simulink model "TEST_TCP"  (R2022b)
settings: Solver=FixedStepAuto  StartTime=0.0  StopTime=inf  FixedStep=1e-3  RelTol=1e-3  EnableMultiTasking=on
undefined symbols (not defined in the file or in its folder): angular, CIRCUIT, CLTF_DAMP, CLTF_FREQ, CLTF_GAIN, CONTROL, CONTROL_INI, DiscIntNeverNeededParam, INPUT, linear, MCP3201, MD25, MODEL, MODEL_INI, mpcstate, MPU60X0, MPU9250, MSG, NAV_MPC_CONTROL, OUTPUT, RCRX, SAMPLING_TIME, SYSID_INPUT, VL6180X
libraries: raspberrypiCommlib x156, simulink x86, dspsigattribs x14, raspberrypiNetworklib x13, embedlinuxBasiclib x9, ctrlSharedLib x2, ros2lib x2, mpclib x1, vrlib x1, sldrtlib x1
(part 3 of 17)

== system TEST_TCP/SIMULATION/READ IMU ==
  " LPF 3" : Subsystem
  " LPF 4" : Subsystem
  ACCEL_X : RandomNumber  Variance=MODEL_INI.PARAM.IMU_ACCEL_NOISE^2  Seed=500  SampleTime=MPU60X0.SAMPLING_TIME
  ACCEL_Y : RandomNumber  Variance=MODEL_INI.PARAM.IMU_ACCEL_NOISE^2  Seed=1000  SampleTime=MPU60X0.SAMPLING_TIME
  ACCEL_Z : RandomNumber  Variance=MODEL_INI.PARAM.IMU_ACCEL_NOISE^2  Seed=2000  SampleTime=MPU60X0.SAMPLING_TIME
  Bus Selector : BusSelector  OutputSignals=OUTPUT.matDCM_BE,OUTPUT.BODY_VEL_DER,OUTPUT.BODY_RATE_DER,OUTPUT.BODY_RATE
  Constant : Constant  Value=[0 0 -MODEL_INI.PARAM.GRAVITY]'  SampleTime=MPU60X0.SAMPLING_TIME
  Constant3 : Constant  Value=CONTROL_INI.PARAM.GRAVITY  SampleTime=MPU60X0.SAMPLING_TIME
  Constant5 : Constant  Value=MPU60X0.ACCEL_CALIB  SampleTime=MPU60X0.SAMPLING_TIME
  Constant6 : Constant  Value=MPU60X0.ALFA_CALIB  SampleTime=MPU60X0.SAMPLING_TIME
  Data Store Memory1 : DataStoreMemory  Priority=10  DataStoreName=MPU60X0_PITCH_OFFS  ReadBeforeWriteMsg=warning  WriteAfterWriteMsg=warning  WriteAfterReadMsg=warning  ShowAdditionalParam=off  OutDataTypeStr=double
  Data Store Memory3 : DataStoreMemory  Priority=10  DataStoreName=MPU60X0_ACCEL_OFFS  ReadBeforeWriteMsg=warning  WriteAfterWriteMsg=warning  WriteAfterReadMsg=warning  InitialValue=zeros(3,1)  ShowAdditionalParam=off  OutDataTypeStr=double
  Data Store Memory4 : DataStoreMemory  Priority=10  DataStoreName=MPU60X0_GYRO_OFFS  ReadBeforeWriteMsg=warning  WriteAfterWriteMsg=warning  WriteAfterReadMsg=warning  InitialValue=zeros(3,1)  ShowAdditionalParam=off  OutDataTypeStr=double
  Data Store Read : DataStoreRead  DataStoreName=CONTROL  DataStoreElements=CONTROL.STATE.VEHICLE_MODE  IndexOptions=Index vector (dialog)  Indices=1  OutputSizes=1
  Data Store Read1 : DataStoreRead  DataStoreName=MPU60X0_ACCEL_OFFS  SampleTime=MPU60X0.SAMPLING_TIME  IndexOptions=Index vector (dialog)  Indices=1  OutputSizes=1
  Data Store Read10 : DataStoreRead  DataStoreName=MODEL  SampleTime=MPU60X0.SAMPLING_TIME  IndexOptions=Index vector (dialog)  Indices=1  OutputSizes=1
  Data Store Read12 : DataStoreRead  DataStoreName=CONTROL  SampleTime=MPU60X0.SAMPLING_TIME  IndexOptions=Index vector (dialog)  Indices=1  OutputSizes=1
  Data Store Read2 : DataStoreRead  DataStoreName=MPU60X0_PITCH_OFFS  SampleTime=MPU60X0.SAMPLING_TIME  IndexOptions=Index vector (dialog)  Indices=1  OutputSizes=1
  Data Store Read4 : DataStoreRead  DataStoreName=MPU60X0_GYRO_OFFS  SampleTime=MPU60X0.SAMPLING_TIME  IndexOptions=Index vector (dialog)  Indices=1  OutputSizes=1
  Data Store Write : DataStoreWrite  DataStoreName=MPU60X0_ACCEL_OFFS  IndexOptions=Index vector (dialog)  Indices=1  OutputSizes=1
  Data Store Write1 : DataStoreWrite  DataStoreName=MPU60X0_GYRO_OFFS  IndexOptions=Index vector (dialog)  Indices=1  OutputSizes=1
  Data Store Write5 : DataStoreWrite  DataStoreName=CONTROL  IndexOptions=Index vector (dialog)  Indices=1  OutputSizes=1
  Divide : Product  Inputs=**  Multiplication=Matrix(*)
  FILTER POLE : Subsystem
  GRAVITY ROTATION : MATLAB Function  TreatAsAtomicUnit=on
  GYRO_X : RandomNumber  Variance=MODEL_INI.PARAM.IMU_GYRO_NOISE^2  Seed=3000  SampleTime=MPU60X0.SAMPLING_TIME
  GYRO_Y : RandomNumber  Variance=MODEL_INI.PARAM.IMU_GYRO_NOISE^2  Seed=4000  SampleTime=MPU60X0.SAMPLING_TIME
  GYRO_Z : RandomNumber  Variance=MODEL_INI.PARAM.IMU_GYRO_NOISE^2  Seed=5000  SampleTime=MPU60X0.SAMPLING_TIME
  Gain1 : Gain  Gain=MODEL_INI.PARAM.NOISE_FLAG
  Gain2 : Gain  Gain=MODEL_INI.PARAM.NOISE_FLAG
  IMU CALIBRATION : MATLAB Function  Priority=30  TreatAsAtomicUnit=on
  LPF 1 : Subsystem
  LPF 2 2 : Subsystem
  MEAN FILTER : DiscreteFilter  Numerator=1/floor(SAMPLING_TIME*1000)*ones(1,floor(SAMPLING_TIME*1000))  Denominator=[1 zeros(1,floor(SAMPLING_TIME*1000)-1)]
  "MEAN FILTER " : DiscreteFilter  Numerator=1/floor(SAMPLING_TIME*1000)*ones(1,floor(SAMPLING_TIME*1000))  Denominator=[1 zeros(1,floor(SAMPLING_TIME*1000)-1)]
  Math Function : Math  Operator=transpose  SignedPower=on
  Mux : Mux  Inputs=3
  Mux1 : Mux  Inputs=3
  Sum : Sum
  Sum1 : Sum  Inputs=++|
  Sum2 : Sum  Inputs=++|
  Terminator : Terminator
  wires:
  Sum1/1 -> IMU CALIBRATION/2(ACCEL), LPF 1/1(IN), MEAN FILTER/1
  MEAN FILTER/1 -> IMU CALIBRATION/4(ACCEL_MEAN), LPF 2 2/1(IN)
  IMU CALIBRATION/2(ACCEL_OFFS_OUT) -> Data Store Write/1
  Sum2/1 -> IMU CALIBRATION/6(GYRO), " LPF 3"/1(IN), "MEAN FILTER "/1
  IMU CALIBRATION/3(GYRO_OFFS_OUT) -> Data Store Write1/1
  Constant5/1 -> IMU CALIBRATION/10(ACCEL_CALIB)
  Constant6/1 -> IMU CALIBRATION/11(ALFA_CALIB)
  "MEAN FILTER "/1 -> IMU CALIBRATION/8(GYRO_MEAN), " LPF 4"/1(IN)
  " LPF 4"/1(OUT) -> IMU CALIBRATION/9(GYRO_MEAN_FILT)
  LPF 2 2/1(OUT) -> IMU CALIBRATION/5(ACCEL_MEAN_FILT)
  Data Store Read12/1 -> IMU CALIBRATION/1(CONTROL_IN)
  IMU CALIBRATION/1(CONTROL) -> Data Store Write5/1
  Mux/1 -> Gain2/1  "GYRO_NOISE"
  ACCEL_X/1 -> Mux1/1
  ACCEL_Y/1 -> Mux1/2
  Mux1/1 -> Gain1/1  "ACCEL_NOISE"
  GYRO_Z/1 -> Mux/3
  ACCEL_Z/1 -> Mux1/3
  GYRO_X/1 -> Mux/1
  GYRO_Y/1 -> Mux/2
  Data Store Read10/1 -> Bus Selector/1
  Bus Selector/1 -> Math Function/1  "<matDCM_BE>"
  Constant/1 -> Divide/2
  Divide/1 -> Sum/1
  Math Function/1 -> Divide/1
  Sum/1 -> Sum1/2
  Bus Selector/4 -> Sum2/1  "<BODY_RATE>"
  Data Store Read1/1 -> IMU CALIBRATION/12(ACCEL_OFFS_IN)
  Data Store Read4/1 -> IMU CALIBRATION/13(GYRO_OFFS_IN)
  Gain2/1 -> Sum2/2
  Bus Selector/2 -> Sum/2  "<BODY_VEL_DER>"
  Bus Selector/3 -> Terminator/1  "<BODY_RATE_DER>"
  FILTER POLE/1(ALFA) -> " LPF 4"/2(ALFA), " LPF 3"/2(ALFA), LPF 1/2(ALFA), LPF 2 2/2(ALFA)
  GRAVITY ROTATION/1(GRAVITY_VECTOR) -> IMU CALIBRATION/14(GRAVITY_VECTOR)
  LPF 1/1(OUT) -> IMU CALIBRATION/3(ACCEL_FILT)
  " LPF 3"/1(OUT) -> IMU CALIBRATION/7(GYRO_FILT)
  Constant3/1 -> GRAVITY ROTATION/2(GRAVITY)
  Data Store Read/1 -> GRAVITY ROTATION/3(VEHICLE_MODE)
  Data Store Read2/1 -> GRAVITY ROTATION/1(PITCH_OFFSET)
  Gain1/1 -> Sum1/1

== system TEST_TCP/CONTROL/LOCAL TARGETS/FORWARD VELOCITY TARGET ==
  Enable : EnablePort
  " PULSE GENERATION" : MATLAB Function  Priority=60  TreatAsAtomicUnit=on
  Bias : Bias  Bias=1  SaturateOnIntegerOverflow=off
  Cast1 : DataTypeConversion  OutDataTypeStr=double  SaturateOnIntegerOverflow=off  RndMeth=Floor
  Compare To Constant : simulink/Logic and Bit Operations/Compare To Constant  relop===  const=0  OutDataTypeStr=boolean
  Compare To Constant1 : simulink/Logic and Bit Operations/Compare To Constant  relop=>=  const=5  OutDataTypeStr=boolean
  Constant : Constant  Value=SYSID_INPUT(:,1)  SampleTime=SAMPLING_TIME
  Constant1 : Constant  Value=0  OutDataTypeStr=double  SampleTime=SAMPLING_TIME
  Constant2 : Constant  Value=0.15  OutDataTypeStr=double  SampleTime=SAMPLING_TIME
  Constant3 : Constant  Value=SAMPLING_TIME  OutDataTypeStr=double  SampleTime=SAMPLING_TIME
  Constant5 : Constant  Value=0.25  OutDataTypeStr=double  SampleTime=SAMPLING_TIME
  Counter Free-Running : simulink/Sources/Counter Free-Running  NumBits=9  tsamp=SAMPLING_TIME
  Data Store Read : DataStoreRead  DataStoreName=CONTROL  SampleTime=SAMPLING_TIME  DataStoreElements=CONTROL.STATE.FV_TARGET_TYPE  IndexOptions=Index vector (dialog)  Indices=1  OutputSizes=1
  Data Store Read1 : DataStoreRead  DataStoreName=CONTROL  SampleTime=SAMPLING_TIME  DataStoreElements=CONTROL.PARAM.OP_OUTPUT(1,:)#CONTROL.PARAM.FV_TARGET_VALUE  IndexOptions=Index vector (dialog)  Indices=1  OutputSizes=1
  Data Store Read2 : DataStoreRead  DataStoreName=CONTROL  SampleTime=SAMPLING_TIME  DataStoreElements=CONTROL.PARAM.OP_OUTPUT(1,:)  IndexOptions=Index vector (dialog)  Indices=1  OutputSizes=1
  Data Store Read3 : DataStoreRead  DataStoreName=CONTROL  SampleTime=SAMPLING_TIME  IndexOptions=Index vector (dialog)  Indices=1  OutputSizes=1
  Data Store Read4 : DataStoreRead  DataStoreName=CONTROL  SampleTime=SAMPLING_TIME  DataStoreElements=CONTROL.STATE.FV_TARGET_TYPE  IndexOptions=Index vector (dialog)  Indices=1  OutputSizes=1
  Data Store Read5 : DataStoreRead  DataStoreName=CONTROL  SampleTime=SAMPLING_TIME  DataStoreElements=CONTROL.PARAM.SAMPLING_TIME  IndexOptions=Index vector (dialog)  Indices=1  OutputSizes=1
  Data Store Read6 : DataStoreRead  DataStoreName=CONTROL  SampleTime=SAMPLING_TIME  DataStoreElements=CONTROL.STATE.VEHICLE_MODE  IndexOptions=Index vector (dialog)  Indices=1  OutputSizes=1
  Data Store Read7 : DataStoreRead  DataStoreName=CONTROL  SampleTime=SAMPLING_TIME  DataStoreElements=CONTROL.STATE.VEHICLE_MODE  IndexOptions=Index vector (dialog)  Indices=1  OutputSizes=1
  Data Store Write1 : DataStoreWrite  DataStoreName=CONTROL  SampleTime=SAMPLING_TIME  DataStoreElements=CONTROL.TARGET.FORWARD_VEL_REF_LC  IndexOptions=Index vector (dialog)  Indices=1  OutputSizes=1
  Data Type Conversion : DataTypeConversion  OutDataTypeStr=double  SaturateOnIntegerOverflow=off  RndMeth=Floor
  Gain2 : Gain  Gain=0.15/2
  Logical Operator : Logic  Operator=OR  AllPortsSameDT=off  OutDataTypeStr=boolean
  Multiport Switch : MultiPortSwitch  DataPortOrder=Zero-based contiguous  Inputs=6  zeroidx=on  SaturateOnIntegerOverflow=off  InputSameDT=off
  Mux : Mux  Inputs=2
  Product : Product
  Pulse Generator1 : DiscretePulseGenerator  Amplitude=0.15  Period=round(10/SAMPLING_TIME)  PulseWidth=round(5/SAMPLING_TIME)  SampleTime=SAMPLING_TIME
  Pulse Generator2 : DiscretePulseGenerator  Amplitude=0.15  Period=round(3/SAMPLING_TIME)  PulseWidth=round(1.5/SAMPLING_TIME)  PhaseDelay=round(0/SAMPLING_TIME)  SampleTime=SAMPLING_TIME
  RAMP : MATLAB Function  TreatAsAtomicUnit=on
  Selector : Selector  IndexMode=Zero-based  InputPortWidth=512  IndexOptions=Index vector (port)  Indices=[1 3]  OutputSizes=1
  Selector1 : Selector  IndexMode=Zero-based  InputPortWidth=5  IndexOptions=Index vector (port)  Indices=[1 3]  OutputSizes=1
  Selector2 : Selector  InputPortWidth=4  IndexOptions=Index vector (port)  Indices=[1 3]  OutputSizes=1
  Sum1 : Sum  Inputs=|++
  Sum3 : Sum  Inputs=|++
  Sum6 : Sum  Inputs=|++
  Switch : Switch  Criteria=u2 > Threshold  Threshold=0.5  SaturateOnIntegerOverflow=off  InputSameDT=off
  Unit Delay : UnitDelay  SampleTime=SAMPLING_TIME  HasFrameUpgradeWarning=on
  wires:
  Constant5/1 -> Sum3/2
  Counter Free-Running/1 -> Cast1/1
  Sum6/1 -> Multiport Switch/5
  Gain2/1 -> Sum6/1
  Selector1/1 -> Multiport Switch/2
  Constant/1 -> Selector/1
  Data Store Read/1 -> Multiport Switch/1
  Cast1/1 -> Selector/2
  Constant2/1 -> Sum6/2
  Multiport Switch/1 -> Data Store Write1/1
  Data Store Read3/1 -> " PULSE GENERATION"/1(CONTROL)
  " PULSE GENERATION"/1(FORWARD_VEL_REF) -> Multiport Switch/3
  Data Store Read1/2 -> Selector1/2
  Selector2/1 -> Multiport Switch/6
  Data Store Read2/1 -> Selector2/1
  Data Store Read4/1 -> Multiport Switch/7
  RAMP/1(ramp_out) -> Selector2/2
  Data Store Read5/1 -> RAMP/1(SAMPLING_TIME)
  Selector/1 -> Bias/1
  Bias/1 -> Gain2/1
  Mux/1 -> Selector1/1
  Data Store Read1/1 -> Mux/2
  Constant1/1 -> Mux/1
  Sum3/1 -> Product/2
  Product/1 -> Multiport Switch/4
  Compare To Constant/1 -> Logical Operator/1
  Data Store Read6/1 -> Compare To Constant/1
  Logical Operator/1 -> Product/1
  Unit Delay/1 -> Sum1/2
  Constant3/1 -> Sum1/1
  Compare To Constant1/1 -> Logical Operator/2
  Sum1/1 -> Compare To Constant1/1, Unit Delay/1
  Data Store Read7/1 -> Data Type Conversion/1
  Switch/1 -> Sum3/1
  Pulse Generator2/1 -> Switch/3
  Pulse Generator1/1 -> Switch/1
  Data Type Conversion/1 -> Switch/2

== system TEST_TCP/CONTROL/LOCAL TARGETS/NAVIGATION TARGETS ==
  Enable : EnablePort
  Constant : Constant  SampleTime=SAMPLING_TIME
  Constant1 : Constant  SampleTime=SAMPLING_TIME
  Data Store Read : DataStoreRead  DataStoreName=CONTROL  SampleTime=SAMPLING_TIME  DataStoreElements=CONTROL.STATE.NAV_TARGET_TYPE(1,1)  IndexOptions=Index vector (dialog)  Indices=1  OutputSizes=1
  Data Store Read2 : DataStoreRead  DataStoreName=CONTROL  SampleTime=SAMPLING_TIME  DataStoreElements=CONTROL.STATE.NAV_TARGET_TYPE(1,2)  IndexOptions=Index vector (dialog)  Indices=1  OutputSizes=1
  Data Store Read4 : DataStoreRead  DataStoreName=CONTROL  SampleTime=SAMPLING_TIME  DataStoreElements=CONTROL.PARAM.NAV_TARGET_VALUE(1,2)  IndexOptions=Index vector (dialog)  Indices=1  OutputSizes=1
  Data Store Read7 : DataStoreRead  Commented=on  DataStoreName=CONTROL  SampleTime=SAMPLING_TIME  IndexOptions=Index vector (dialog)  Indices=1  OutputSizes=1
  Data Store Read9 : DataStoreRead  DataStoreName=CONTROL  SampleTime=SAMPLING_TIME  DataStoreElements=CONTROL.PARAM.NAV_TARGET_VALUE(1,1)  IndexOptions=Index vector (dialog)  Indices=1  OutputSizes=1
  Data Store Write : DataStoreWrite  Commented=on  DataStoreName=CONTROL  SampleTime=SAMPLING_TIME  IndexOptions=Index vector (dialog)  Indices=1  OutputSizes=1
  Data Store Write1 : DataStoreWrite  DataStoreName=CONTROL  SampleTime=SAMPLING_TIME  DataStoreElements=CONTROL.TARGET.NAV_REF_LC(1,1)  IndexOptions=Index vector (dialog)  Indices=1  OutputSizes=1
  Data Store Write2 : DataStoreWrite  DataStoreName=CONTROL  SampleTime=SAMPLING_TIME  DataStoreElements=CONTROL.TARGET.NAV_REF_LC(2,1)  IndexOptions=Index vector (dialog)  Indices=1  OutputSizes=1
  Multiport Switch : MultiPortSwitch  DataPortOrder=Zero-based contiguous  Inputs=4  zeroidx=on  SaturateOnIntegerOverflow=off  InputSameDT=off
  Multiport Switch1 : MultiPortSwitch  DataPortOrder=Zero-based contiguous  Inputs=4  zeroidx=on  SaturateOnIntegerOverflow=off  InputSameDT=off
  PATH PLANNER : MATLAB Function  Priority=10  Commented=on  TreatAsAtomicUnit=on
  Pulse Generator1 : DiscretePulseGenerator  Amplitude=2  Period=round(50/SAMPLING_TIME)  PulseWidth=round(25/SAMPLING_TIME)  PhaseDelay=round(12.5/SAMPLING_TIME)  SampleTime=SAMPLING_TIME
  Pulse Generator2 : DiscretePulseGenerator  Amplitude=2  Period=round(50/SAMPLING_TIME)  PulseWidth=round(25/SAMPLING_TIME)  SampleTime=SAMPLING_TIME
  Sine Wave : Sin  SineType=Sample based  Samples=round(40/SAMPLING_TIME)  SampleTime=SAMPLING_TIME
  Sine Wave1 : Sin  SineType=Sample based  Samples=round(40/SAMPLING_TIME)  SampleTime=SAMPLING_TIME  Offset=round(30/SAMPLING_TIME)
  Sum1 : Sum  Inputs=|+-
  Sum3 : Sum  Inputs=|+-
  TRAJECTORY PLANNER (POLYNOMIAL IN Vx & Vy) : MATLAB Function  Priority=10  Commented=on  TreatAsAtomicUnit=on
  wires:
  Data Store Read7/1 -> TRAJECTORY PLANNER (POLYNOMIAL IN Vx & Vy)/1(CONTROL_IN)
  TRAJECTORY PLANNER (POLYNOMIAL IN Vx & Vy)/1(CONTROL) -> Data Store Write/1
  Data Store Read/1 -> Multiport Switch/1
  Multiport Switch/1 -> Data Store Write1/1
  Sum3/1 -> Multiport Switch/5, Multiport Switch/3
  Data Store Read9/1 -> Multiport Switch/2
  Sine Wave/1 -> Multiport Switch/4
  Data Store Read4/1 -> Multiport Switch1/2
  Data Store Read2/1 -> Multiport Switch1/1
  Sine Wave1/1 -> Multiport Switch1/4
  Multiport Switch1/1 -> Data Store Write2/1
  Sum1/1 -> Multiport Switch1/5, Multiport Switch1/3
  Pulse Generator2/1 -> Sum3/1
  Constant/1 -> Sum3/2
  Pulse Generator1/1 -> Sum1/1
  Constant1/1 -> Sum1/2

== system TEST_TCP/CONTROL/LOCAL TARGETS/OPL TARGETS ==
  Enable : EnablePort
  Cast : DataTypeConversion  OutDataTypeStr=uint8  SaturateOnIntegerOverflow=off  RndMeth=Floor
  Cast1 : DataTypeConversion  OutDataTypeStr=double  SaturateOnIntegerOverflow=off  RndMeth=Floor
  Constant : Constant  Value=SYSID_INPUT(:,1)  SampleTime=SAMPLING_TIME
  Constant1 : Constant  Value=SYSID_INPUT(:,2)  SampleTime=SAMPLING_TIME
  Constant2 : Constant  Value=2  OutDataTypeStr=single  SampleTime=SAMPLING_TIME
  Constant3 : Constant  Value=2  OutDataTypeStr=double  SampleTime=SAMPLING_TIME
  Constant5 : Constant  Value=4  OutDataTypeStr=double  SampleTime=SAMPLING_TIME
  Constant6 : Constant  Value=0  OutDataTypeStr=double  SampleTime=SAMPLING_TIME
  Constant7 : Constant  Value=-0.25  OutDataTypeStr=single  SampleTime=SAMPLING_TIME
  Constant8 : Constant  Value=2  OutDataTypeStr=double  SampleTime=SAMPLING_TIME
  Counter Free-Running : simulink/Sources/Counter Free-Running  NumBits=9  tsamp=SAMPLING_TIME
  Counter Free-Running1 : simulink/Sources/Counter Free-Running  NumBits=9  tsamp=SAMPLING_TIME
  Data Store Read : DataStoreRead  DataStoreName=CONTROL  SampleTime=SAMPLING_TIME  DataStoreElements=CONTROL.STATE.MV_TARGET_TYPE(1,1)  IndexOptions=Index vector (dialog)  Indices=1  OutputSizes=1
  Data Store Read1 : DataStoreRead  DataStoreName=CONTROL  SampleTime=SAMPLING_TIME  IndexOptions=Index vector (dialog)  Indices=1  OutputSizes=1
  Data Store Read2 : DataStoreRead  DataStoreName=CONTROL  SampleTime=SAMPLING_TIME  DataStoreElements=CONTROL.STATE.MV_TARGET_TYPE(2,1)  IndexOptions=Index vector (dialog)  Indices=1  OutputSizes=1
  Data Store Write1 : DataStoreWrite  DataStoreName=CONTROL  SampleTime=SAMPLING_TIME  DataStoreElements=CONTROL.TARGET.MOTOR_VOLT_CD_REF_LC(:,:)  IndexOptions=Index vector (dialog)  Indices=1  OutputSizes=1
  Gain2 : Gain
  Gain3 : Gain
  Multiport Switch : MultiPortSwitch  DataPortOrder=Zero-based contiguous  Inputs=4  zeroidx=on  SaturateOnIntegerOverflow=off  InputSameDT=off
  Multiport Switch1 : MultiPortSwitch  DataPortOrder=Zero-based contiguous  Inputs=4  zeroidx=on  SaturateOnIntegerOverflow=off  InputSameDT=off
  Mux : Mux  Inputs=2
  Pulse Generator1 : DiscretePulseGenerator  Amplitude=2  Period=200  PulseWidth=100  SampleTime=SAMPLING_TIME
  Pulse Generator3 : DiscretePulseGenerator  Amplitude=2  Period=200  PulseWidth=100  SampleTime=SAMPLING_TIME
  Selector : Selector  IndexMode=Zero-based  InputPortWidth=512  IndexOptions=Index vector (port)  Indices=[1 3]  OutputSizes=1
  Selector1 : Selector  IndexMode=Zero-based  InputPortWidth=512  IndexOptions=Index vector (port)  Indices=[1 3]  OutputSizes=1
  Sum{1,3,6,8} (4 alike) : Sum  Inputs=|++
  VOLTAGE PULSE GENERATION : MATLAB Function  Priority=60  TreatAsAtomicUnit=on
  wires:
  VOLTAGE PULSE GENERATION/1(MOTOR_VOLT_TARGET) -> Multiport Switch/3, Multiport Switch1/3
  Constant6/1 -> Multiport Switch1/2
  Constant7/1 -> Sum8/2
  Sum6/1 -> Multiport Switch/5
  Mux/1 -> Data Store Write1/1
  Sum3/1 -> Multiport Switch/4
  Gain2/1 -> Sum6/1
  Counter Free-Running/1 -> Cast1/1
  Cast1/1 -> Selector/2
  Sum8/1 -> Multiport Switch1/5
  Sum1/1 -> Multiport Switch1/4
  Selector1/1 -> Gain3/1
  Multiport Switch1/1 -> Mux/2
  Constant1/1 -> Selector1/1
  Constant/1 -> Selector/1
  Gain3/1 -> Sum8/1
  Multiport Switch/1 -> Mux/1
  Data Store Read2/1 -> Multiport Switch1/1
  Cast/1 -> Selector1/2
  Constant2/1 -> Sum6/2
  Selector/1 -> Gain2/1
  Counter Free-Running1/1 -> Cast/1
  Data Store Read/1 -> Multiport Switch/1
  Data Store Read1/1 -> VOLTAGE PULSE GENERATION/1(CONTROL)
  Constant5/1 -> Multiport Switch/2
  Pulse Generator1/1 -> Sum3/1
  Constant3/1 -> Sum3/2
  Pulse Generator3/1 -> Sum1/1
  Constant8/1 -> Sum1/2

== system TEST_TCP/CONTROL/LOCAL TARGETS/WFL TARGETS ==
  Enable : EnablePort
  " PULSE GENERATION" : MATLAB Function  Priority=60  TreatAsAtomicUnit=on
  Cast1 : DataTypeConversion  OutDataTypeStr=double  SaturateOnIntegerOverflow=off  RndMeth=Floor
  Compare To Constant : simulink/Logic and Bit Operations/Compare To Constant  relop=<=  const=3.0  OutDataTypeStr=uint8
  Constant : Constant  Value=SYSID_INPUT(:,1)  SampleTime=SAMPLING_TIME
  Constant1 : Constant  Value=0.1  OutDataTypeStr=double  SampleTime=SAMPLING_TIME
  Constant3 : Constant  Value=0.25  OutDataTypeStr=double  SampleTime=SAMPLING_TIME
  Constant5 : Constant  Value=0.025  OutDataTypeStr=single  SampleTime=SAMPLING_TIME
  Counter Free-Running : simulink/Sources/Counter Free-Running  NumBits=9  tsamp=SAMPLING_TIME
  Data Store Read : DataStoreRead  DataStoreName=CONTROL  SampleTime=SAMPLING_TIME  DataStoreElements=CONTROL.STATE.WD_TARGET_TYPE  IndexOptions=Index vector (dialog)  Indices=1  OutputSizes=1
  Data Store Read1 : DataStoreRead  DataStoreName=CONTROL  SampleTime=SAMPLING_TIME  DataStoreElements=CONTROL.STATE.WALL_FOLLOWER_MODE  IndexOptions=Index vector (dialog)  Indices=1  OutputSizes=1
  Data Store Read3 : DataStoreRead  DataStoreName=CONTROL  SampleTime=SAMPLING_TIME  IndexOptions=Index vector (dialog)  Indices=1  OutputSizes=1
  Data Store Write1 : DataStoreWrite  DataStoreName=CONTROL  SampleTime=SAMPLING_TIME  DataStoreElements=CONTROL.TARGET.WALL_DIST_REF_LC  IndexOptions=Index vector (dialog)  Indices=1  OutputSizes=1
  Data Type Conversion : DataTypeConversion  OutDataTypeStr=double  SaturateOnIntegerOverflow=off  RndMeth=Floor
  Gain2 : Gain  Gain=0.025
  Multiport Switch : MultiPortSwitch  DataPortOrder=Zero-based contiguous  Inputs=4  zeroidx=on  SaturateOnIntegerOverflow=off  InputSameDT=off
  Product : Product
  Pulse Generator1 : DiscretePulseGenerator  Amplitude=0.025  Period=1000  PulseWidth=500  SampleTime=SAMPLING_TIME
  Selector : Selector  IndexMode=Zero-based  InputPortWidth=512  IndexOptions=Index vector (port)  Indices=[1 3]  OutputSizes=1
  Sum3 : Sum  Inputs=+|+|-
  Sum6 : Sum  Inputs=|++
  Switch : Switch  Criteria=u2 > Threshold  Threshold=0.5  SaturateOnIntegerOverflow=off  InputSameDT=off
  wires:
  Data Store Read3/1 -> " PULSE GENERATION"/1(CONTROL)
  Sum6/1 -> Multiport Switch/5
  Sum3/1 -> Multiport Switch/4
  Constant/1 -> Selector/1
  " PULSE GENERATION"/1(WALL_DIST_REF) -> Multiport Switch/3
  Switch/1 -> Sum6/2, Sum3/1, Multiport Switch/2
  Gain2/1 -> Sum6/1
  Multiport Switch/1 -> Data Store Write1/1
  Cast1/1 -> Selector/2
  Selector/1 -> Gain2/1
  Counter Free-Running/1 -> Cast1/1
  Product/1 -> Multiport Switch/1
  Data Store Read/1 -> Compare To Constant/1, Product/1
  Compare To Constant/1 -> Product/2
  Constant3/1 -> Switch/1
  Constant1/1 -> Switch/3
  Pulse Generator1/1 -> Sum3/2
  Constant5/1 -> Sum3/3
  Data Store Read1/1 -> Data Type Conversion/1
  Data Type Conversion/1 -> Switch/2

== system TEST_TCP/CONTROL/LOCAL TARGETS/YAW ANGLE TARGET ==
  Enable : EnablePort
  " PULSE GENERATION" : MATLAB Function  Priority=60  TreatAsAtomicUnit=on
  Cast1 : DataTypeConversion  OutDataTypeStr=double  SaturateOnIntegerOverflow=off  RndMeth=Floor
  Constant : Constant  Value=SYSID_INPUT(:,1)  SampleTime=SAMPLING_TIME
  Constant3 : Constant  Value=0  OutDataTypeStr=double  SampleTime=SAMPLING_TIME
  Constant5 : Constant  Value=-60*pi/180  OutDataTypeStr=single  SampleTime=SAMPLING_TIME
  Constant8 : Constant  Value=-60*pi/180  OutDataTypeStr=single  SampleTime=SAMPLING_TIME
  Counter Free-Running : simulink/Sources/Counter Free-Running  NumBits=9  tsamp=SAMPLING_TIME
  Data Store Read : DataStoreRead  DataStoreName=CONTROL  SampleTime=SAMPLING_TIME  DataStoreElements=CONTROL.STATE.YA_TARGET_TYPE  IndexOptions=Index vector (dialog)  Indices=1  OutputSizes=1
  Data Store Read1 : DataStoreRead  DataStoreName=CONTROL  SampleTime=SAMPLING_TIME  IndexOptions=Index vector (dialog)  Indices=1  OutputSizes=1
  Data Store Write1 : DataStoreWrite  DataStoreName=CONTROL  SampleTime=SAMPLING_TIME  DataStoreElements=CONTROL.TARGET.YAW_ANG_REF_LC  IndexOptions=Index vector (dialog)  Indices=1  OutputSizes=1
  Gain2 : Gain  Gain=120*pi/180
  Multiport Switch : MultiPortSwitch  DataPortOrder=Zero-based contiguous  Inputs=4  zeroidx=on  SaturateOnIntegerOverflow=off  InputSameDT=off
  Pulse Generator1 : DiscretePulseGenerator  Amplitude=120*pi/180  Period=500  PulseWidth=250  PhaseDelay=125  SampleTime=SAMPLING_TIME
  Selector : Selector  IndexMode=Zero-based  InputPortWidth=512  IndexOptions=Index vector (port)  Indices=[1 3]  OutputSizes=1
  Sum3 : Sum  Inputs=|++
  Sum6 : Sum  Inputs=|++
  wires:
  Constant5/1 -> Sum3/2
  Selector/1 -> Gain2/1
  Pulse Generator1/1 -> Sum3/1
  Counter Free-Running/1 -> Cast1/1
  Sum6/1 -> Multiport Switch/5
  " PULSE GENERATION"/1(YAW_ANG_REF) -> Multiport Switch/3
  Sum3/1 -> Multiport Switch/4
  Gain2/1 -> Sum6/1
  Constant3/1 -> Multiport Switch/2
  Constant/1 -> Selector/1
  Data Store Read/1 -> Multiport Switch/1
  Data Store Read1/1 -> " PULSE GENERATION"/1(CONTROL)
  Cast1/1 -> Selector/2
  Constant8/1 -> Sum6/2
  Multiport Switch/1 -> Data Store Write1/1

== system TEST_TCP/CONTROL/LOCAL TARGETS/YAW RATE TARGET ==
  Enable : EnablePort
  " PULSE GENERATION " : MATLAB Function  Priority=60  TreatAsAtomicUnit=on
  Bias : Bias  Bias=1  SaturateOnIntegerOverflow=off
  Cast : DataTypeConversion  OutDataTypeStr=uint8  SaturateOnIntegerOverflow=off  RndMeth=Floor
  Constant1 : Constant  Value=SYSID_INPUT(:,2)  SampleTime=SAMPLING_TIME
  Constant6 : Constant  Value=0  OutDataTypeStr=double  SampleTime=SAMPLING_TIME
  Constant8 : Constant  Value=-60*pi/180  OutDataTypeStr=single  SampleTime=SAMPLING_TIME
  Constant9 : Constant  Value=-60*pi/180  OutDataTypeStr=single  SampleTime=SAMPLING_TIME
  Counter Free-Running1 : simulink/Sources/Counter Free-Running  NumBits=9  tsamp=SAMPLING_TIME
  Data Store Read1 : DataStoreRead  DataStoreName=CONTROL  SampleTime=SAMPLING_TIME  IndexOptions=Index vector (dialog)  Indices=1  OutputSizes=1
  Data Store Read2 : DataStoreRead  DataStoreName=CONTROL  SampleTime=SAMPLING_TIME  DataStoreElements=CONTROL.STATE.YR_TARGET_TYPE  IndexOptions=Index vector (dialog)  Indices=1  OutputSizes=1
  Data Store Write2 : DataStoreWrite  DataStoreName=CONTROL  SampleTime=SAMPLING_TIME  DataStoreElements=CONTROL.TARGET.YAW_RATE_REF_LC  IndexOptions=Index vector (dialog)  Indices=1  OutputSizes=1
  Gain1 : Gain  Gain=60*pi/180
  Multiport Switch1 : MultiPortSwitch  DataPortOrder=Zero-based contiguous  Inputs=4  zeroidx=on  SaturateOnIntegerOverflow=off  InputSameDT=off
  Pulse Generator2 : DiscretePulseGenerator  Amplitude=120*pi/180  Period=round(3/SAMPLING_TIME)  PulseWidth=round(1.5/SAMPLING_TIME)  PhaseDelay=round(0.75/SAMPLING_TIME)  SampleTime=SAMPLING_TIME
  Selector1 : Selector  IndexMode=Zero-based  InputPortWidth=512  IndexOptions=Index vector (port)  Indices=[1 3]  OutputSizes=1
  Sum1 : Sum  Inputs=|++
  Sum2 : Sum  Inputs=|++
  wires:
  Sum2/1 -> Multiport Switch1/5
  Data Store Read2/1 -> Multiport Switch1/1
  Constant1/1 -> Selector1/1
  Multiport Switch1/1 -> Data Store Write2/1
  Constant6/1 -> Multiport Switch1/2
  Counter Free-Running1/1 -> Cast/1
  Cast/1 -> Selector1/2
  Data Store Read1/1 -> " PULSE GENERATION "/1(CONTROL)
  " PULSE GENERATION "/1(YAW_RATE_REF) -> Multiport Switch1/3
  Constant8/1 -> Sum1/2
  Constant9/1 -> Sum2/2
  Pulse Generator2/1 -> Sum1/1
  Selector1/1 -> Bias/1
  Sum1/1 -> Multiport Switch1/4
  Gain1/1 -> Sum2/1
  Bias/1 -> Gain1/1

== system TEST_TCP/CONTROL/SYSTEM IDENTIFICATION/FILTER TIME CONSTANT ==
  Enable : EnablePort
  Constant5 : Constant  Value=0.05  OutDataTypeStr=single  SampleTime=SAMPLING_TIME
  Data Store Write1 : DataStoreWrite  DataStoreName=CONTROL  SampleTime=SAMPLING_TIME  DataStoreElements=CONTROL.PARAM.ENC_FILT_FREQ  IndexOptions=Index vector (dialog)  Indices=1  OutputSizes=1
  Data Store Write2 : DataStoreWrite  DataStoreName=CONTROL  SampleTime=SAMPLING_TIME  DataStoreElements=CONTROL.PARAM.FILT_TIME_CONSTANT_ACT  IndexOptions=Index vector (dialog)  Indices=1  OutputSizes=1
  Gain : Gain  Gain=1/2/pi
  Math Function : Math  Operator=reciprocal
  Pulse Generator1 : DiscretePulseGenerator  Amplitude=0.05  Period=16000  PulseWidth=8000  PhaseDelay=8000  SampleTime=SAMPLING_TIME
  Sum3 : Sum  Inputs=|++
  wires:
  Pulse Generator1/1 -> Sum3/1
  Constant5/1 -> Sum3/2
  Sum3/1 -> Data Store Write2/1, Math Function/1
  Math Function/1 -> Gain/1
  Gain/1 -> Data Store Write1/1

== system TEST_TCP/CONTROL/SYSTEM IDENTIFICATION/STATE VARIABLE FILTER 1 ==
  IN : Inport
  Add : Sum  Inputs=3
  Constant : Constant  Value=SVF_B1d  SampleTime=SAMPLING_TIME
  Constant1 : Constant  Value=SVF_B2d  SampleTime=SAMPLING_TIME
  Constant2 : Constant  Value=SVF_Ad  SampleTime=SAMPLING_TIME
  Divide : Product  Multiplication=Matrix(*)
  Divide1 : Product  Multiplication=Matrix(*)
  Divide2 : Product  Multiplication=Matrix(*)
  Unit Delay : UnitDelay  InitialCondition=zeros(4,1)  SampleTime=-1  HasFrameUpgradeWarning=on
  Unit Delay1 : UnitDelay  SampleTime=-1  HasFrameUpgradeWarning=on
  STATE : Outport  VectorParamsAs1DForOutWhenUnconnected=off
  wires:
  Constant/1 -> Divide1/1
  Unit Delay1/1 -> Divide1/2
  Divide1/1 -> Add/1
  Add/1 -> STATE/1, Unit Delay/1
  Divide/1 -> Add/2
  Constant1/1 -> Divide/1
  Divide2/1 -> Add/3
  Constant2/1 -> Divide2/1
  Unit Delay/1 -> Divide2/2
  IN/1 -> Divide/2, Unit Delay1/1

== system TEST_TCP/CONTROL/SYSTEM IDENTIFICATION/STATE VARIABLE FILTER 2 ==
  IN : Inport
  Add : Sum  Inputs=3
  Constant : Constant  Value=SVF_B1d  SampleTime=SAMPLING_TIME
  Constant1 : Constant  Value=SVF_B2d  SampleTime=SAMPLING_TIME
  Constant2 : Constant  Value=SVF_Ad  SampleTime=SAMPLING_TIME
  Divide : Product  Multiplication=Matrix(*)
  Divide1 : Product  Multiplication=Matrix(*)
  Divide2 : Product  Multiplication=Matrix(*)
  Unit Delay : UnitDelay  InitialCondition=zeros(4,1)  SampleTime=-1  HasFrameUpgradeWarning=on
  Unit Delay1 : UnitDelay  SampleTime=-1  HasFrameUpgradeWarning=on
  STATE : Outport  VectorParamsAs1DForOutWhenUnconnected=off
  wires:
  IN/1 -> Unit Delay1/1, Divide/2
  Unit Delay/1 -> Divide2/2
  Constant2/1 -> Divide2/1
  Divide2/1 -> Add/3
  Constant1/1 -> Divide/1
  Divide/1 -> Add/2
  Add/1 -> Unit Delay/1, STATE/1
  Divide1/1 -> Add/1
  Unit Delay1/1 -> Divide1/2
  Constant/1 -> Divide1/1

== system TEST_TCP/CONTROL/SYSTEM IDENTIFICATION/STATE VARIABLE FILTER 3 ==
  IN : Inport
  Add : Sum  Inputs=3
  Constant : Constant  Value=SVF_B1d  SampleTime=SAMPLING_TIME
  Constant1 : Constant  Value=SVF_B2d  SampleTime=SAMPLING_TIME
  Constant2 : Constant  Value=SVF_Ad  SampleTime=SAMPLING_TIME
  Divide : Product  Multiplication=Matrix(*)
  Divide1 : Product  Multiplication=Matrix(*)
  Divide2 : Product  Multiplication=Matrix(*)
  Unit Delay : UnitDelay  InitialCondition=zeros(4,1)  SampleTime=-1  HasFrameUpgradeWarning=on
  Unit Delay1 : UnitDelay  SampleTime=-1  HasFrameUpgradeWarning=on
  STATE : Outport  VectorParamsAs1DForOutWhenUnconnected=off
  wires:
  Constant/1 -> Divide1/1
  Unit Delay1/1 -> Divide1/2
  Divide1/1 -> Add/1
  Add/1 -> STATE/1, Unit Delay/1
  Divide/1 -> Add/2
  Constant1/1 -> Divide/1
  Divide2/1 -> Add/3
  Constant2/1 -> Divide2/1
  Unit Delay/1 -> Divide2/2
  IN/1 -> Divide/2, Unit Delay1/1

== system TEST_TCP/CONTROL/SYSTEM IDENTIFICATION/STATE VARIABLE FILTER 4 ==
  IN : Inport
  Add : Sum  Inputs=3
  Constant : Constant  Value=SVF_B1d  SampleTime=SAMPLING_TIME
  Constant1 : Constant  Value=SVF_B2d  SampleTime=SAMPLING_TIME
  Constant2 : Constant  Value=SVF_Ad  SampleTime=SAMPLING_TIME
  Divide : Product  Multiplication=Matrix(*)
  Divide1 : Product  Multiplication=Matrix(*)
  Divide2 : Product  Multiplication=Matrix(*)
  Unit Delay : UnitDelay  InitialCondition=zeros(4,1)  SampleTime=-1  HasFrameUpgradeWarning=on
  Unit Delay1 : UnitDelay  SampleTime=-1  HasFrameUpgradeWarning=on
  STATE : Outport  VectorParamsAs1DForOutWhenUnconnected=off
  wires:
  IN/1 -> Unit Delay1/1, Divide/2
  Unit Delay/1 -> Divide2/2
  Constant2/1 -> Divide2/1
  Divide2/1 -> Add/3
  Constant1/1 -> Divide/1
  Divide/1 -> Add/2
  Add/1 -> Unit Delay/1, STATE/1
  Divide1/1 -> Add/1
  Unit Delay1/1 -> Divide1/2
  Constant/1 -> Divide1/1

== system TEST_TCP/HARDWARE/ACTUATORS/MD25_I2C ==
  Cast : DataTypeConversion  OutDataTypeStr=uint8  SaturateOnIntegerOverflow=off  RndMeth=Floor
  Compare To Constant : simulink/Logic and Bit Operations/Compare To Constant  relop===  const=0  OutDataTypeStr=uint8
  Data Store Memory : DataStoreMemory  Priority=10  DataStoreName=MD25_INIT  ReadBeforeWriteMsg=warning  WriteAfterWriteMsg=warning  WriteAfterReadMsg=warning  ShowAdditionalParam=off  OutDataTypeStr=boolean
  Data Store Read : DataStoreRead  DataStoreName=MD25_INIT  SampleTime=SAMPLING_TIME  IndexOptions=Index vector (dialog)  Indices=1  OutputSizes=1
  Data Store Read1 : DataStoreRead  DataStoreName=MD25_INIT  IndexOptions=Index vector (dialog)  Indices=1  OutputSizes=1
  Data Store Read2 : DataStoreRead  DataStoreName=CONTROL  SampleTime=SAMPLING_TIME  DataStoreElements=CONTROL.STATE.CURRENT_STATUS_SYS  IndexOptions=Index vector (dialog)  Indices=1  OutputSizes=1
  Data Store Write : DataStoreWrite  DataStoreName=CONTROL  DataStoreElements=CONTROL.STATE.MD25_INIT  IndexOptions=Index vector (dialog)  Indices=1  OutputSizes=1
  Logical Operator : Logic  Operator=NOT  AllPortsSameDT=off  OutDataTypeStr=boolean
  MD25 INITIALIZATION : Subsystem  Priority=10
      settings: RTWSystemCode=Nonreusable function
  READ BATTERY VOLTAGE : Subsystem  Priority=20  TreatAsAtomicUnit=on
      settings: RTWSystemCode=Nonreusable function
  READ MOTOR CURRENT : Subsystem  Priority=30  TreatAsAtomicUnit=on
      settings: RTWSystemCode=Nonreusable function
  READ MOTOR ENCODER : Subsystem  Priority=40  TreatAsAtomicUnit=on
      settings: RTWSystemCode=Nonreusable function
  RESET MOTOR ENCODER : Subsystem  Priority=50  TreatAsAtomicUnit=on
      settings: RTWSystemCode=Nonreusable function
  "WRITE PWM MOTOR " : Subsystem  Priority=50  TreatAsAtomicUnit=on
      settings: RTWSystemCode=Nonreusable function
  wires:
  Logical Operator/1 -> MD25 INITIALIZATION/Enable
  Data Store Read1/1 -> Cast/1
  Cast/1 -> Data Store Write/1
  Data Store Read/1 -> "WRITE PWM MOTOR "/Enable, READ MOTOR ENCODER/Enable, READ MOTOR CURRENT/Enable, READ BATTERY VOLTAGE/Enable, Logical Operator/1
  Data Store Read2/1 -> Compare To Constant/1
  Compare To Constant/1 -> RESET MOTOR ENCODER/Enable

== system TEST_TCP/HARDWARE/ACTUATORS/RGB ==
  BLUE : embedlinuxBasiclib/GPIO Write  board=Pi 3 Model B+  gpio=25  direction=Output  blockPlatform=Raspberry Pi
  Cast1 : DataTypeConversion  OutDataTypeStr=boolean  SaturateOnIntegerOverflow=off  RndMeth=Floor
  Cast2 : DataTypeConversion  OutDataTypeStr=boolean  SaturateOnIntegerOverflow=off  RndMeth=Floor
  Cast3 : DataTypeConversion  OutDataTypeStr=boolean  SaturateOnIntegerOverflow=off  RndMeth=Floor
  Data Store Read : DataStoreRead  DataStoreName=CONTROL  SampleTime=SAMPLING_TIME  DataStoreElements=CONTROL.OUTPUT.LEDS(:,:)  IndexOptions=Index vector (dialog)  Indices=1  OutputSizes=1
  Demux : Demux  Outputs=3
  GREEN : embedlinuxBasiclib/GPIO Write  board=Pi 3 Model B+  gpio=24  direction=Output  blockPlatform=Raspberry Pi
  RED : embedlinuxBasiclib/GPIO Write  board=Pi 3 Model B+  gpio=23  direction=Output  blockPlatform=Raspberry Pi
  wires:
  Data Store Read/1 -> Demux/1
  Demux/1 -> Cast1/1
  Demux/2 -> Cast2/1
  Demux/3 -> Cast3/1
  Cast1/1 -> RED/1
  Cast2/1 -> GREEN/1
  Cast3/1 -> BLUE/1

== system TEST_TCP/HARDWARE/COMMUNICATIONS/BT_RX ==
  Bus Selector : BusSelector  OutputSignals=INPUT.MCS_EARTH_POS,INPUT.MCS_EULER_ANG
  Data Store Read2 : DataStoreRead  DataStoreName=CONTROL  SampleTime=SAMPLING_TIME  IndexOptions=Index vector (dialog)  Indices=1  OutputSizes=1
  Data Store Write1 : DataStoreWrite  DataStoreName=CONTROL  DataStoreElements=CONTROL.STATE.MCS_RX_STATUS  IndexOptions=Index vector (dialog)  Indices=1  OutputSizes=1
  Data Store Write2 : DataStoreWrite  DataStoreName=CONTROL  IndexOptions=Index vector (dialog)  Indices=1  OutputSizes=1
  Data Type Conversion : DataTypeConversion  OutDataTypeStr=uint8  SaturateOnIntegerOverflow=off  RndMeth=Floor
  Display{,1..3} (4 alike) : Display
  MCS RX : MATLAB Function  Priority=20  TreatAsAtomicUnit=on
  MCS_EARTH_POS : Scope
  MCS_EULER_ANG : Scope
  Serial Read : raspberrypiCommlib/Serial Read  board=Pi 3 Model B+  SCIModule_=/dev/ttyUSB0  Baudrate_=115200  Parity=None  StopBits_=1  HardwareFlowControl=None  ByteOrder=LittleEndian  DataLength=50  DataType=uint8  OutputStatus=on  SampleTime=SAMPLING_TIME  blockPlatform=RaspberryPi
  wires:
  MCS RX/1(CONTROL) -> Bus Selector/1, Data Store Write2/1
  Data Store Read2/1 -> MCS RX/1(CONTROL_IN)
  Serial Read/1 -> Display1/1, MCS RX/2(BUFFER_RX_LAST)
  Serial Read/2 -> Data Type Conversion/1
  Bus Selector/1 -> MCS_EARTH_POS/1, Display2/1  "<MCS_EARTH_POS>"
  Bus Selector/2 -> MCS_EULER_ANG/1, Display3/1  "<MCS_EULER_ANG>"
  Data Type Conversion/1 -> Data Store Write1/1, Display/1, MCS RX/3(STATUS)

== system TEST_TCP/HARDWARE/COMMUNICATIONS/TCP//IP ==
  Compare To Zero : simulink/Logic and Bit Operations/Compare To Zero  relop=>  OutDataTypeStr=boolean
  Data Store Read : DataStoreRead  DataStoreName=MSG  SampleTime=SAMPLING_TIME  DataStoreElements=MSG.TX_BUFFER(1,1)  IndexOptions=Index vector (dialog)  Indices=1  OutputSizes=1
  MSG_RX : Subsystem  Priority=10  TreatAsAtomicUnit=on
      settings: RTWSystemCode=Nonreusable function  FunctionWithSeparateData=on
  MSG_TX : Subsystem  Priority=10
      settings: RTWSystemCode=Nonreusable function  FunctionWithSeparateData=on
  wires:
  Compare To Zero/1 -> MSG_TX/Enable
  Data Store Read/1 -> Compare To Zero/1

== system TEST_TCP/HARDWARE/COMMUNICATIONS/TCP//IP LIDAR ==
  Bus Selector : BusSelector  OutputSignals=INPUT.LIDAR_2D
  Data Store Read1 : DataStoreRead  DataStoreName=CONTROL  SampleTime=SAMPLING_TIME  DataStoreElements=CONTROL.STATE.LIDAR_2D_MODE  IndexOptions=Index vector (dialog)  Indices=1  OutputSizes=1
  Data Store Read2 : DataStoreRead  DataStoreName=CONTROL  SampleTime=SAMPLING_TIME  IndexOptions=Index vector (dialog)  Indices=1  OutputSizes=1
  Data Store Write1 : DataStoreWrite  DataStoreName=CONTROL  DataStoreElements=CONTROL.STATE.NAV_RX_STATUS  IndexOptions=Index vector (dialog)  Indices=1  OutputSizes=1
  Data Store Write2 : DataStoreWrite  DataStoreName=CONTROL  IndexOptions=Index vector (dialog)  Indices=1  OutputSizes=1
  Data Type Conversion : DataTypeConversion  OutDataTypeStr=uint8  SaturateOnIntegerOverflow=off  RndMeth=Floor
  Display : Display
  Display1 : Display
  Display2 : Display
  NAV RX : MATLAB Function  Priority=20  TreatAsAtomicUnit=on
  TCP/IP Receive : raspberrypiNetworklib/TCP//IP Receive  Mode_=Server  LocalServerPort_=7000  RemoteAddr_=127.0.0.1  RemoteServerPort_=3000  DataType_=uint8  DataSize_=160  SampleTime_=SAMPLING_TIME  SimulateUsing=Code generation  ClientPortBindingSelection_=off  ClientPortToBind_=35000  BlockingMode_=off  BlockTimeout_=0.1  BlockPlatform=RASPBERRYPI
  TCP/IP Send : raspberrypiNetworklib/TCP//IP Send  Mode_=Server  LocalServerPort_=7001  RemoteAddr_=127.0.0.1  RemoteServerPort_=25000  SimulateUsing=Code generation  ClientPortBindingSelection_=off  ClientPortToBind_=35000  BlockingMode_=off  BlockTimeout_=0.1  BlockPlatform=RASPBERRYPI
  wires:
  NAV RX/1(CONTROL) -> Bus Selector/1, Data Store Write2/1
  Data Store Read2/1 -> NAV RX/1(CONTROL_IN)
  TCP/IP Receive/1 -> NAV RX/2(PAYLOAD), Display1/1
  Bus Selector/1 -> Display2/1  "<LIDAR_2D>"
  Data Type Conversion/1 -> Data Store Write1/1, Display/1, NAV RX/3(STATUS)
  TCP/IP Receive/2 -> Data Type Conversion/1
  Data Store Read1/1 -> TCP/IP Send/1

== system TEST_TCP/HARDWARE/COMMUNICATIONS/TCP//IP MCS ==
  Bus Selector : BusSelector  OutputSignals=INPUT.MCS_EARTH_POS,INPUT.MCS_EULER_ANG
  Data Store Read2 : DataStoreRead  DataStoreName=CONTROL  SampleTime=SAMPLING_TIME  IndexOptions=Index vector (dialog)  Indices=1  OutputSizes=1
  Data Store Write1 : DataStoreWrite  DataStoreName=CONTROL  DataStoreElements=CONTROL.STATE.MCS_RX_STATUS  IndexOptions=Index vector (dialog)  Indices=1  OutputSizes=1
  Data Store Write2 : DataStoreWrite  DataStoreName=CONTROL  IndexOptions=Index vector (dialog)  Indices=1  OutputSizes=1
  Data Type Conversion : DataTypeConversion  OutDataTypeStr=uint8  SaturateOnIntegerOverflow=off  RndMeth=Floor
  Display{,1..3} (4 alike) : Display
  MCS RX : MATLAB Function  Priority=20  TreatAsAtomicUnit=on
  MCS_EARTH_POS : Scope
  MCS_EULER_ANG : Scope
  TCP/IP Receive : raspberrypiNetworklib/TCP//IP Receive  Mode_=Server  LocalServerPort_=15000  RemoteAddr_=127.0.0.1  RemoteServerPort_=3000  DataType_=uint8  DataSize_=26  SampleTime_=SAMPLING_TIME  SimulateUsing=Code generation  ClientPortBindingSelection_=off  ClientPortToBind_=35000  BlockingMode_=off  BlockTimeout_=0.1  BlockPlatform=RASPBERRYPI
  wires:
  TCP/IP Receive/2 -> Data Type Conversion/1
  Data Type Conversion/1 -> MCS RX/3(STATUS), Display/1, Data Store Write1/1
  Bus Selector/2 -> Display3/1, MCS_EULER_ANG/1  "<MCS_EULER_ANG>"
  Bus Selector/1 -> Display2/1, MCS_EARTH_POS/1  "<MCS_EARTH_POS>"
  TCP/IP Receive/1 -> Display1/1, MCS RX/2(PAYLOAD)
  Data Store Read2/1 -> MCS RX/1(CONTROL_IN)
  MCS RX/1(CONTROL) -> Data Store Write2/1, Bus Selector/1

== system TEST_TCP/HARDWARE/COMMUNICATIONS/TCP//IP NAV ==
  Bus Selector : BusSelector  OutputSignals=INPUT.NAV_EARTH_POS,INPUT.NAV_EULER_ANG
  Data Store Read2 : DataStoreRead  DataStoreName=CONTROL  SampleTime=SAMPLING_TIME  IndexOptions=Index vector (dialog)  Indices=1  OutputSizes=1
  Data Store Write1 : DataStoreWrite  DataStoreName=CONTROL  DataStoreElements=CONTROL.STATE.NAV_RX_STATUS  IndexOptions=Index vector (dialog)  Indices=1  OutputSizes=1
  Data Store Write2 : DataStoreWrite  DataStoreName=CONTROL  IndexOptions=Index vector (dialog)  Indices=1  OutputSizes=1
  Data Type Conversion : DataTypeConversion  OutDataTypeStr=uint8  SaturateOnIntegerOverflow=off  RndMeth=Floor
  Display{,1..3} (4 alike) : Display
  NAV RX : MATLAB Function  Priority=20  TreatAsAtomicUnit=on
  NAV_EARTH_POS : Scope
  NAV_EULER_ANG : Scope
  TCP/IP Receive : raspberrypiNetworklib/TCP//IP Receive  Mode_=Server  LocalServerPort_=3000  RemoteAddr_=127.0.0.1  RemoteServerPort_=3000  DataType_=uint8  DataSize_=24  SampleTime_=SAMPLING_TIME  SimulateUsing=Code generation  ClientPortBindingSelection_=off  ClientPortToBind_=35000  BlockingMode_=off  BlockTimeout_=0.1  BlockPlatform=RASPBERRYPI
  wires:
  NAV RX/1(CONTROL) -> Bus Selector/1, Data Store Write2/1
  Data Store Read2/1 -> NAV RX/1(CONTROL_IN)
  TCP/IP Receive/1 -> NAV RX/2(PAYLOAD), Display1/1
  Bus Selector/1 -> NAV_EARTH_POS/1, Display2/1  "<NAV_EARTH_POS>"
  Bus Selector/2 -> NAV_EULER_ANG/1, Display3/1  "<NAV_EULER_ANG>"
  Data Type Conversion/1 -> Data Store Write1/1, Display/1, NAV RX/3(STATUS)
  TCP/IP Receive/2 -> Data Type Conversion/1

== system TEST_TCP/HARDWARE/COMMUNICATIONS/TCP//IP RPI4 ==
  Bus Selector : BusSelector  OutputSignals=INPUT.LIDAR_2D,TARGET.NAV_REF_PC
  Data Store Read2 : DataStoreRead  DataStoreName=CONTROL  SampleTime=SAMPLING_TIME  IndexOptions=Index vector (dialog)  Indices=1  OutputSizes=1
  Data Store Read3 : DataStoreRead  DataStoreName=CONTROL  SampleTime=SAMPLING_TIME  IndexOptions=Index vector (dialog)  Indices=1  OutputSizes=1
  Data Store Write1 : DataStoreWrite  DataStoreName=CONTROL  DataStoreElements=CONTROL.STATE.NAV_RX_STATUS  IndexOptions=Index vector (dialog)  Indices=1  OutputSizes=1
  Data Store Write2 : DataStoreWrite  DataStoreName=CONTROL  IndexOptions=Index vector (dialog)  Indices=1  OutputSizes=1
  Data Type Conversion : DataTypeConversion  OutDataTypeStr=uint8  SaturateOnIntegerOverflow=off  RndMeth=Floor
  Display{,1..3} (4 alike) : Display
  RPI4 CODER : MATLAB Function  Priority=20  TreatAsAtomicUnit=on
  RPI4 DECODER : MATLAB Function  Priority=20  TreatAsAtomicUnit=on
  Scope : Scope
  TCP/IP Receive : raspberrypiNetworklib/TCP//IP Receive  Mode_=Server  LocalServerPort_=7000  RemoteAddr_=127.0.0.1  RemoteServerPort_=3000  DataType_=uint8  DataSize_=1064  SampleTime_=SAMPLING_TIME  SimulateUsing=Code generation  ClientPortBindingSelection_=off  ClientPortToBind_=35000  BlockingMode_=off  BlockTimeout_=0.1  BlockPlatform=RASPBERRYPI
  TCP/IP Send : raspberrypiNetworklib/TCP//IP Send  Mode_=Server  LocalServerPort_=7001  RemoteAddr_=127.0.0.1  RemoteServerPort_=25000  SimulateUsing=Code generation  ClientPortBindingSelection_=off  ClientPortToBind_=35000  BlockingMode_=off  BlockTimeout_=0.1  BlockPlatform=RASPBERRYPI
  wires:
  TCP/IP Receive/2 -> Data Type Conversion/1
  Data Type Conversion/1 -> RPI4 DECODER/3(STATUS), Display/1, Data Store Write1/1
  Bus Selector/1 -> Display2/1  "<LIDAR_2D>"
  TCP/IP Receive/1 -> RPI4 DECODER/2(RX_MSG), Display1/1
  Data Store Read2/1 -> RPI4 DECODER/1(CONTROL_IN)
  RPI4 DECODER/1(CONTROL) -> Bus Selector/1, Data Store Write2/1
  Data Store Read3/1 -> RPI4 CODER/1(CONTROL)
  Bus Selector/2 -> Scope/1  "<NAV_REF_PC>"
  RPI4 CODER/1(TX_MSG) -> Display3/1, TCP/IP Send/1

== system TEST_TCP/HARDWARE/COMMUNICATIONS/TCP//IP SLAM ==
  Data Store Read1 : DataStoreRead  DataStoreName=CONTROL  SampleTime=SAMPLING_TIME  IndexOptions=Index vector (dialog)  Indices=1  OutputSizes=1
  SLAM TX : MATLAB Function  Priority=20  TreatAsAtomicUnit=on
  TCP/IP Send : raspberrypiNetworklib/TCP//IP Send  Mode_=Server  LocalServerPort_=7001  RemoteAddr_=127.0.0.1  RemoteServerPort_=25000  SimulateUsing=Code generation  ClientPortBindingSelection_=off  ClientPortToBind_=35000  BlockingMode_=off  BlockTimeout_=0.1  BlockPlatform=RASPBERRYPI
  wires:
  SLAM TX/1(PAYLOAD) -> TCP/IP Send/1
  Data Store Read1/1 -> SLAM TX/1(CONTROL)

== system TEST_TCP/HARDWARE/COMMUNICATIONS/TCP//IP TEST ==
  Constant : Constant  Value=127  OutDataTypeStr=uint8  SampleTime=SAMPLING_TIME
  Data Type Conversion : DataTypeConversion  OutDataTypeStr=uint8  SaturateOnIntegerOverflow=off  RndMeth=Floor
  Display2 : Display
  Display3 : Display
  TCP/IP Receive : raspberrypiNetworklib/TCP//IP Receive  Mode_=Client  LocalServerPort_=3000  RemoteAddr_=192.168.1.21  RemoteServerPort_=27000  DataType_=uint8  DataSize_=1  SampleTime_=SAMPLING_TIME  SimulateUsing=Code generation  ClientPortBindingSelection_=off  ClientPortToBind_=35000  BlockingMode_=off  BlockTimeout_=0.1  BlockPlatform=RASPBERRYPI
  TCP/IP Send : raspberrypiNetworklib/TCP//IP Send  Mode_=Server  LocalServerPort_=27000  RemoteAddr_=127.0.0.1  RemoteServerPort_=25000  SimulateUsing=Code generation  ClientPortBindingSelection_=off  ClientPortToBind_=35000  BlockingMode_=off  BlockTimeout_=0.1  BlockPlatform=RASPBERRYPI
  wires:
  TCP/IP Receive/2 -> Data Type Conversion/1
  Data Type Conversion/1 -> Display3/1
  Constant/1 -> TCP/IP Send/1
  TCP/IP Receive/1 -> Display2/1

== system TEST_TCP/HARDWARE/COMMUNICATIONS/UART ==
  Compare To Zero : simulink/Logic and Bit Operations/Compare To Zero  relop=>  OutDataTypeStr=boolean
  Data Store Read : DataStoreRead  DataStoreName=CONTROL  SampleTime=SAMPLING_TIME  DataStoreElements=CONTROL.STATE.UART_MODE  IndexOptions=Index vector (dialog)  Indices=1  OutputSizes=1
  MSG_RX : Subsystem  Priority=10
      settings: RTWSystemCode=Nonreusable function  FunctionWithSeparateData=on
  MSG_TX : Subsystem  Priority=10
      settings: RTWSystemCode=Nonreusable function  FunctionWithSeparateData=on
  wires:
  Data Store Read/1 -> Compare To Zero/1
  Compare To Zero/1 -> MSG_TX/Enable

== system TEST_TCP/HARDWARE/COMMUNICATIONS/UART_MUX ==
  A : embedlinuxBasiclib/GPIO Write  Priority=4  board=Pi 3 Model B+  gpio=8  direction=Output  blockPlatform=Raspberry Pi
  B : embedlinuxBasiclib/GPIO Write  Priority=5  board=Pi 3 Model B+  gpio=18  direction=Output  blockPlatform=Raspberry Pi
  BT MCS : Subsystem  Priority=1
      settings: RTWSystemCode=Nonreusable function  FunctionWithSeparateData=on
  INH : embedlinuxBasiclib/GPIO Write  Priority=6  board=Pi 3 Model B+  gpio=5  direction=Output  blockPlatform=Raspberry Pi
  MATLAB Function : MATLAB Function  Priority=3  TreatAsAtomicUnit=on
  RCRX iBUS : Subsystem  Priority=2
  Serial Read : raspberrypiCommlib/Serial Read  Priority=0  board=Pi 3 Model B+  SCIModule_=/dev/ttyS0  Baudrate_=57600  Parity=None  StopBits_=1  HardwareFlowControl=None  ByteOrder=LittleEndian  DataLength=50  DataType=uint8  OutputStatus=on  SampleTime=SAMPLING_TIME  blockPlatform=RaspberryPi
  Terminator : Terminator
  wires:
  Serial Read/1 -> BT MCS/1(Data), RCRX iBUS/1(Data)
  Serial Read/2 -> Terminator/1
  MATLAB Function/5(BL) -> BT MCS/Enable
  MATLAB Function/4(RCRX) -> RCRX iBUS/Enable
  MATLAB Function/3(INH) -> INH/1
  MATLAB Function/2(B) -> B/1
  MATLAB Function/1(A) -> A/1

== system TEST_TCP/HARDWARE/COMMUNICATIONS/UDP//ROS ==
  Compare To Zero : simulink/Logic and Bit Operations/Compare To Zero  relop=>  OutDataTypeStr=boolean
  Data Store Read : DataStoreRead  DataStoreName=MSG  SampleTime=SAMPLING_TIME  DataStoreElements=MSG.TX_BUFFER(1,1)  IndexOptions=Index vector (dialog)  Indices=1  OutputSizes=1
  MSG_RX : Subsystem  Priority=10  TreatAsAtomicUnit=on
      settings: RTWSystemCode=Nonreusable function  FunctionWithSeparateData=on
  MSG_TX : Subsystem  Priority=10
      settings: RTWSystemCode=Nonreusable function  FunctionWithSeparateData=on
  wires:
  Compare To Zero/1 -> MSG_TX/Enable
  Data Store Read/1 -> Compare To Zero/1
